simulink subsystem "Prova_4"  (R2024b)
settings: Solver=VariableStepAuto  StartTime=0.0  StopTime=10.0  RelTol=1e-3
settings Model: Creator=sabpi  LastModifiedBy=sabpi

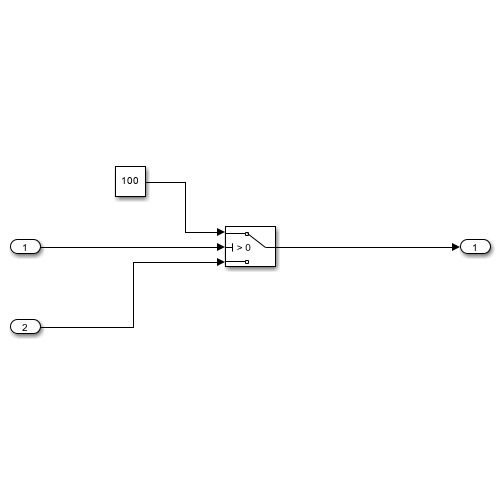
[thumbnail: Simulink's stored preview of the top-level diagram]
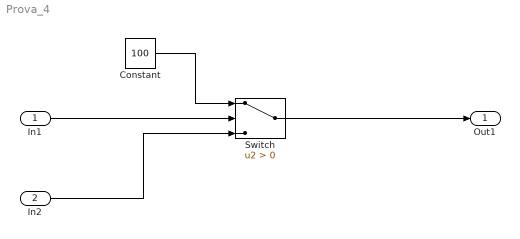
== system Prova_4 ==
  In1 : Inport
  In2 : Inport  Port=2
  Constant : Constant  Value=100
  Switch : Switch  Criteria=u2 > Threshold  SaturateOnIntegerOverflow=off  InputSameDT=off
  Out1 : Outport
  wires:
  In2/1 -> Switch/3
  In1/1 -> Switch/2
  Constant/1 -> Switch/1
  Switch/1 -> Out1/1
